simulink model "model_equation"  (R2021a)
settings: Solver=FixedStepAuto  StartTime=0.0  StopTime=10.0  FixedStep=Ts  RelTol=1e-3
undefined symbols (not defined in the file): acc_C, acc_enable, acc_noise_var, B_hs, b_large_bot, b_large_up, b_small_bot, b_small_up, bot_damp_start, C_1, C_2, C_A_in, C_A_out, C_adj_in, C_adj_out, C_B_in, C_B_out, cycle, F_c, F_df, F_sf, flow_C, flow_C_ratio, flow_noise_var, g, gamma, gn, gp, K_hs, k_small_bot, k_small_up, L, LargeDamper_bottom, LargeDamper_upper, M, M_L, p0, p1, p2, p3, p4, P_0, p_A0, p_B0, P_cr, P_s, prox_bot_band, prox_up_band, R, S_0, S_A, S_B, sg_C, sg_enable, sg_noise_var, SmallDamper_bottom, SmallDamper_upper, spool_dynamic, spool_valve_time_delay, T ... (+6)
settings Model: OrderedModelArguments=off  Creator=artof  LastModifiedBy=artof
settings DataIOCC: ExternalInput=[t, u1, u2]  LoadExternalInput=on

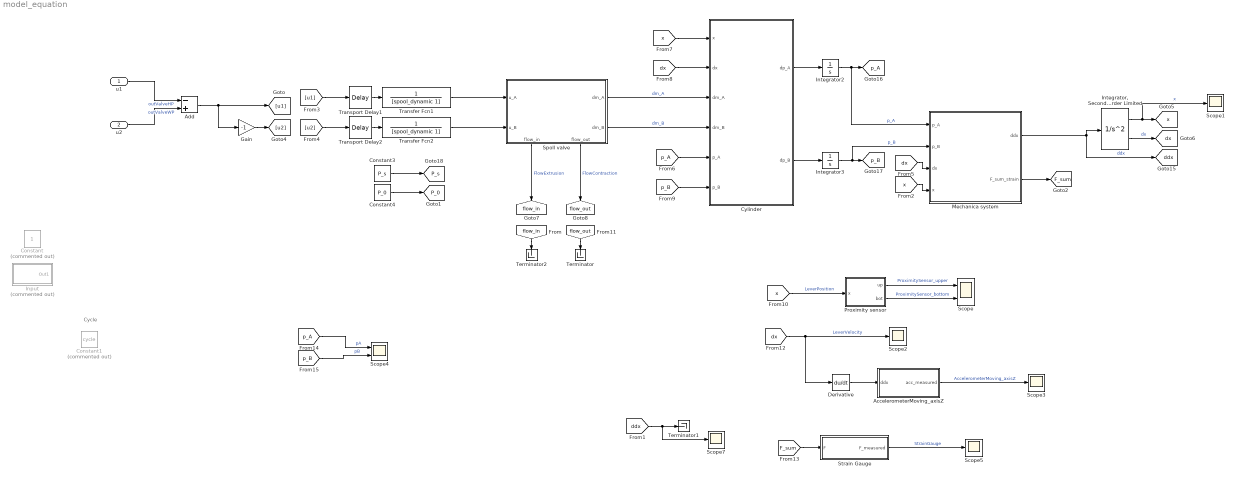
== system model_equation ==
  note: Cycle
  u1 : Inport
  u2 : Inport  Port=2
  AccelerometerMoving_axisZ : MATLAB Function  TreatAsAtomicUnit=on
  Add : Sum  Inputs=-+
  Constant : Constant  Commented=on
  Constant1 : Constant  Commented=on  Value=cycle  VectorParams1D=off  OutDataTypeStr=double
  Constant3 : Constant  Value=P_s
  Constant4 : Constant  Value=P_0
  Cylinder : MATLAB Function  TreatAsAtomicUnit=on
  Derivative : Derivative
  Gain : Gain  Gain=-1
  Input : Subsystem  Commented=on
  "Integrator, Second-Order Limited" : SecondOrderIntegrator  ICX=x0  UpperLimitX=gp  LowerLimitX=gn
  Integrator2 : Integrator  InitialCondition=p_A0
  Integrator3 : Integrator  InitialCondition=p_B0
  Mechanica system : MATLAB Function  TreatAsAtomicUnit=on
  Proximity sensor : MATLAB Function  TreatAsAtomicUnit=on
  Scope : Scope  NumInputPorts=2
  Scope{1..3,5,7} (5 alike) : Scope
  Scope4 : Scope  NumInputPorts=2
  Spoll valve : Subsystem
      settings: PortSchema="{\"entries\":[{\"content\":{\"sides\":[{\"content\":{\"connectorIds\":[\"In1\",\"In2\"]},\"type\":\"ConnectorPlacement.EquallySpacedRectSide\",\"uuid\":\"f49fadee-fa9e-4c00-be17-3013d1757a7f\"},{\"content\":{\"connectorIds\":[\"Out1\",\"Out2\"],\"side\":\"RIGHT\"},\"type\":\"ConnectorPlacement.EquallySpacedRectSide\",\"uuid\":\"640b0073-0df7-45c7-9e72-cb244187d5a1\"},{\"content\":{\"connectorIds\":[],\"side\":\"TOP\"},\"type\":\"ConnectorPlacement.EquallySpacedRectSide\",\"uuid\":\"42e207d6-f026-4ddf-97dc-8c7968fc41f1\"},{\"content\":{\"connectorIds\":[\"Out3\",\"Out4\"],\"side\":\"BOTTOM\"},\"type\":\"ConnectorPlacement.EquallySpacedRectSide\",\"uuid\":\"eeba3cdd-6d70-46a7-a1e2-c2998fe430fd\"}]},\"type\":\"ConnectorPlacement.EquallySpacedConnector\",\"uuid\":\"e8c5a427-dc83-42b8-9540-729b85904a46\"}],\"packageUris\":[\"http://schema.mathworks.com/mf0/Connector/R2020b\"],\"version\":\"1.0\"}"
  Strain Gauge : MATLAB Function  TreatAsAtomicUnit=on
  Terminator : Terminator
  Terminator1 : Terminator
  Terminator2 : Terminator
  Transfer Fcn1 : TransferFcn  Denominator=[spool_dynamic 1]
  Transfer Fcn2 : TransferFcn  Denominator=[spool_dynamic 1]
  Transport Delay1 : TransportDelay  DelayTime=spool_valve_time_delay
  Transport Delay2 : TransportDelay  DelayTime=spool_valve_time_delay
  tag scope: F_sum=global, P_0=global, P_s=global, ddx=global, dx=global, flow_in=global, flow_out=global, p_A=global, p_B=global, x=global
  wires:
  Integrator2/1 -> Mechanica system/1(p_A), [p_A]  "p_A"
  Transport Delay2/1 -> Transfer Fcn2/1
  u1/1 -> Add/1  "outValveHP"
  "Integrator, Second-Order Limited"/1 -> Scope1/1, [x]  "x"
  [x] -> Mechanica system/4(x)
  Proximity sensor/2(bot) -> Scope/2  "ProximitySensor_bottom"
  [flow_out] -> Terminator/1
  Proximity sensor/1(up) -> Scope/1  "ProximitySensor_upper"
  [u2] -> Transport Delay2/1
  Transfer Fcn2/1 -> Spoll valve/2(u_B)
  Spoll valve/1(dm_A) -> Cylinder/3(dm_A)  "dm_A"
  Transfer Fcn1/1 -> Spoll valve/1(u_A)
  [ddx] -> Scope7/1, Terminator1/1
  [p_A] -> Cylinder/5(p_A)
  Spoll valve/4(flow_out) -> [flow_out]  "FlowContraction"
  [F_sum] -> Strain Gauge/1(F)
  Strain Gauge/1(F_measured) -> Scope5/1  "StrainGauge"
  Spoll valve/2(dm_B) -> Cylinder/4(dm_B)  "dm_B"
  [flow_in] -> Terminator2/1
  Mechanica system/1(ddx) -> "Integrator, Second-Order Limited"/1, [ddx]  "ddx"
  Integrator3/1 -> Mechanica system/2(p_B), [p_B]  "p_B"
  Constant3/1 -> [P_s]
  [dx] -> Derivative/1, Scope2/1  "LeverVelocity"
  Transport Delay1/1 -> Transfer Fcn1/1
  Gain/1 -> [u2]
  Constant4/1 -> [P_0]
  Cylinder/1(dp_A) -> Integrator2/1
  Mechanica system/2(F_sum_strain) -> [F_sum]
  [p_B] -> Cylinder/6(p_B)
  Derivative/1 -> AccelerometerMoving_axisZ/1(ddx)
  [dx] -> Mechanica system/3(dx)
  [u1] -> Transport Delay1/1
  AccelerometerMoving_axisZ/1(acc_measured) -> Scope3/1  "AccelerometerMoving_axisZ"
  Cylinder/2(dp_B) -> Integrator3/1
  [dx] -> Cylinder/2(dx)
  [x] -> Cylinder/1(x)
  Spoll valve/3(flow_in) -> [flow_in]  "FlowExtrusion"
  Add/1 -> Gain/1, [u1]
  "Integrator, Second-Order Limited"/2 -> [dx]  "dx"
  [x] -> Proximity sensor/1(x)  "LeverPosition"
  u2/1 -> Add/2  "outValveWP"
  [p_B] -> Scope4/2  "pB"
  [p_A] -> Scope4/1  "pA"

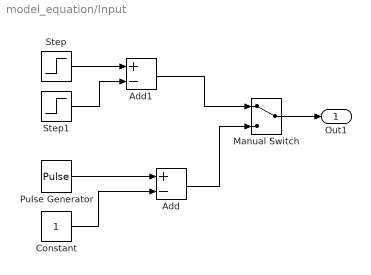
== system model_equation/Input ==
  Add : Sum  Inputs=+-
  Add1 : Sum  Inputs=+-
  Constant : Constant
  Manual Switch : ManualSwitch
  Pulse Generator : DiscretePulseGenerator  PulseType=Time based  Amplitude=2  Period=10  PulseWidth=50
  Step : Step  Before=-1  SampleTime=0
  Step1 : Step  Time=6  After=2  SampleTime=0
  Out1 : Outport
  wires:
  Manual Switch/1 -> Out1/1
  Add/1 -> Manual Switch/2
  Add1/1 -> Manual Switch/1
  Pulse Generator/1 -> Add/1
  Constant/1 -> Add/2
  Step1/1 -> Add1/2
  Step/1 -> Add1/1

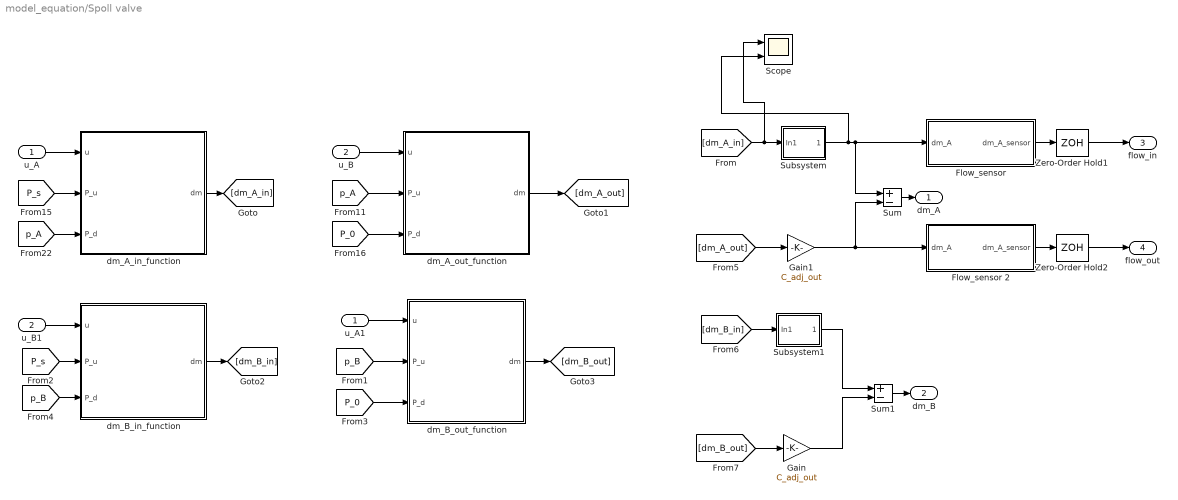
== system model_equation/Spoll valve ==
  u_A : Inport
  u_B : Inport  Port=2
  Flow_sensor : MATLAB Function  TreatAsAtomicUnit=on
  Flow_sensor 2 : MATLAB Function  TreatAsAtomicUnit=on
  Gain : Gain  Gain=C_adj_out
  Gain1 : Gain  Gain=C_adj_out
  Scope : Scope  NumInputPorts=2
  Subsystem : Subsystem
  Subsystem1 : Subsystem
  Sum : Sum  Inputs=+-
  Sum1 : Sum  Inputs=+-
  Zero-Order Hold1 : ZeroOrderHold  SampleTime=Ts
  Zero-Order Hold2 : ZeroOrderHold  SampleTime=Ts
  dm_A_in_function : MATLAB Function  TreatAsAtomicUnit=on
  dm_A_out_function : MATLAB Function  TreatAsAtomicUnit=on
  dm_B_in_function : MATLAB Function  TreatAsAtomicUnit=on
  dm_B_out_function : MATLAB Function  TreatAsAtomicUnit=on
  u_A1 : InportShadow
  u_B1 : InportShadow  Port=2
  dm_A : Outport
  dm_B : Outport  Port=2
  flow_in : Outport  Port=3
  flow_out : Outport  Port=4
  wires:
  [P_s] -> dm_A_in_function/2(P_u)
  [p_A] -> dm_A_in_function/3(P_d)
  dm_A_in_function/1(dm) -> [dm_A_in]
  dm_A_out_function/1(dm) -> [dm_A_out]
  [p_A] -> dm_A_out_function/2(P_u)
  [P_0] -> dm_A_out_function/3(P_d)
  u_A/1 -> dm_A_in_function/1(u)
  u_B/1 -> dm_A_out_function/1(u)
  u_B1/1 -> dm_B_in_function/1(u)
  [P_0] -> dm_B_out_function/3(P_d)
  [p_B] -> dm_B_out_function/2(P_u)
  [p_B] -> dm_B_in_function/3(P_d)
  [P_s] -> dm_B_in_function/2(P_u)
  u_A1/1 -> dm_B_out_function/1(u)
  dm_B_in_function/1(dm) -> [dm_B_in]
  dm_B_out_function/1(dm) -> [dm_B_out]
  [dm_A_in] -> Subsystem/1(In1), Scope/1
  Sum/1 -> dm_A/1
  Sum1/1 -> dm_B/1
  [dm_B_out] -> Gain/1
  [dm_B_in] -> Subsystem1/1(In1)
  Flow_sensor/1(dm_A_sensor) -> Zero-Order Hold1/1
  Flow_sensor 2/1(dm_A_sensor) -> Zero-Order Hold2/1
  [dm_A_out] -> Gain1/1
  Zero-Order Hold1/1 -> flow_in/1
  Zero-Order Hold2/1 -> flow_out/1
  Subsystem1/1(Out1) -> Sum1/1
  Subsystem/1(Out1) -> Scope/2, Sum/1, Flow_sensor/1(dm_A)
  Gain/1 -> Sum1/2
  Gain1/1 -> Flow_sensor 2/1(dm_A), Sum/2

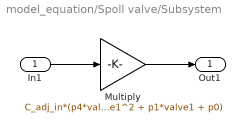
== system model_equation/Spoll valve/Subsystem ==
  In1 : Inport
  Multiply : Gain  Gain=C_adj_in*(p4*valve1^4 + p3*valve1^3+p2*valve1^2 + p1*valve1 + p0)
  Out1 : Outport
  wires:
  In1/1 -> Multiply/1
  Multiply/1 -> Out1/1

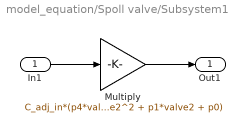
== system model_equation/Spoll valve/Subsystem1 ==
  In1 : Inport
  Multiply : Gain  Gain=C_adj_in*(p4*valve2^4 + p3*valve2^3+p2*valve2^2 + p1*valve2 + p0)
  Out1 : Outport
  wires:
  Multiply/1 -> Out1/1
  In1/1 -> Multiply/1

== matlab function model_equation/Cylinder ==
  data: x input; dp_A output size=1; dx input; dm_A input; dm_B input; p_A input; p_B input; gamma parameter; V_0A parameter; V_0B parameter; S_A parameter; S_B parameter; R parameter; T parameter; dp_B output size=1; L parameter
function [dp_A,dp_B]= fcn(x,dx,dm_A,dm_B,p_A,p_B,gamma,V_0A,V_0B,S_A,S_B,R,T,L)
V_A = V_0A + S_A*x;
dV_A = dx * S_A;

V_B = V_0B + S_B*(L-x);
dV_B = - dx * S_B;

dp_A = dm_A*gamma*R*T/V_A - p_A*gamma*dV_A/V_A;
dp_B = dm_B*gamma*R*T/V_B - p_B*gamma*dV_B/V_B;
end

== matlab function model_equation/Spoll valve/dm_A_in_function ==
  data: u input; dm output; P_u input; P_d input; C_A_in parameter; C_1 parameter; C_2 parameter; P_cr parameter; T parameter; gamma parameter
function dm = fcn(u, P_u, P_d, C_A_in, C_1, C_2, P_cr, T, gamma)
if u > 0    
    P_ratio = P_d/P_u;
    if P_ratio <= P_cr && P_ratio >= 0
        dm = u*C_A_in*C_1*P_u/sqrt(T);
    elseif P_ratio > P_cr && P_ratio <= 1
        dm = u*C_A_in*C_2*P_u/sqrt(T)*P_ratio^(1/gamma)*sqrt(1-P_ratio^((gamma-1)/gamma));
    else
        %dm = -u*C_A_in*C_2*P_d/sqrt(T)*(1/P_ratio)^(1/gamma)*sqrt(1-(1/P_ratio)^((gamma-1)/gamma));
        dm = 0;
    end
else
    dm = 0;
end

== matlab function model_equation/Spoll valve/dm_A_out_function ==
  data: u input; dm output; P_u input; P_d input; C_A_out parameter; C_1 parameter; P_cr parameter; C_2 parameter; T parameter; gamma parameter
function dm = fcn(u, P_u, P_d, C_A_out, C_1, P_cr, C_2, T, gamma)
if u > 0    
    P_ratio = P_d/P_u;
    if P_ratio <= P_cr && P_ratio >= 0
        dm = u*C_A_out*C_1*P_u/sqrt(T);
    elseif P_ratio > P_cr && P_ratio <= 1
        dm = u*C_A_out*C_2*P_u/sqrt(T)*P_ratio^(1/gamma)*sqrt(1-P_ratio^((gamma-1)/gamma));
    else
        %dm = -u*C_A_out*C_2*P_d/sqrt(T)*(1/P_ratio)^(1/gamma)*sqrt(1-(1/P_ratio)^((gamma-1)/gamma));
        dm = 0;
    end
else
    dm = 0;
end

== matlab function model_equation/Spoll valve/dm_B_in_function ==
  data: u input; dm output; P_u input; P_d input; P_cr parameter; C_B_in parameter; C_1 parameter; C_2 parameter; T parameter; gamma parameter
function dm = fcn(u, P_u, P_d, P_cr, C_B_in, C_1, C_2, T, gamma)
if u > 0    
    P_ratio = P_d/P_u;
    if P_ratio <= P_cr && P_ratio >= 0
        dm = u*C_B_in*C_1*P_u/sqrt(T);
    elseif P_ratio > P_cr && P_ratio <= 1
        dm = u*C_B_in*C_2*P_u/sqrt(T)*P_ratio^(1/gamma)*sqrt(1-P_ratio^((gamma-1)/gamma));
    else
        %dm = -u*C_B_in*C_2*P_d/sqrt(T)*(1/P_ratio)^(1/gamma)*sqrt(1-(1/P_ratio)^((gamma-1)/gamma));
        dm = 0;
    end
else
    dm = 0;
end

== matlab function model_equation/Spoll valve/dm_B_out_function ==
  data: u input; dm output; P_u input; P_d input; P_cr parameter; C_B_out parameter; C_1 parameter; C_2 parameter; T parameter; gamma parameter
function dm = fcn(u, P_u, P_d, P_cr, C_B_out, C_1, C_2, T, gamma)
if u > 0    
    P_ratio = P_d/P_u;
    if P_ratio <= P_cr && P_ratio >= 0
        dm = u*C_B_out*C_1*P_u/sqrt(T);
    elseif P_ratio > P_cr && P_ratio <= 1
        dm = u*C_B_out*C_2*P_u/sqrt(T)*P_ratio^(1/gamma)*sqrt(1-P_ratio^((gamma-1)/gamma));
    else
        %dm = -u*C_B_out*C_2*P_d/sqrt(T)*(1/P_ratio)^(1/gamma)*sqrt(1-(1/P_ratio)^((gamma-1)/gamma));
        dm = 0;
    end
else
    dm = 0;
end

== matlab function model_equation/AccelerometerMoving_axisZ ==
  settings: updateMethod=DISCRETE  sampleTime=Ts
  data: ddx input; acc_measured output; acc_noise_var parameter; acc_enable parameter; acc_C parameter
function acc_measured = fcn(ddx, acc_noise_var, acc_enable, acc_C)

ZeroOffset = 2.5; % V
Sensetivity = 333; %mv/g

acc = acc_enable * acc_C * ddx + 1;

U_raw = acc*Sensetivity/1000 + ZeroOffset;
U_raw = U_raw + acc_noise_var*(2*rand()-1);

acc_measured =  acc_enable*((U_raw - ZeroOffset)*1000/Sensetivity);
end

== matlab function model_equation/Proximity sensor ==
  data: x input; up output; bot output; prox_up_band parameter; prox_bot_band parameter
function [up,bot]= fcn(x, prox_up_band, prox_bot_band)
if x >= prox_up_band
    up = 1; bot = 0;
elseif x <= prox_bot_band
    bot = 1; up = 0;
else
    bot = 0;
    up = 0;
end

== matlab function model_equation/Spoll valve/Flow_sensor ==
  settings: updateMethod=DISCRETE
  data: dm_A input; dm_A_sensor output; flow_C parameter; flow_C_ratio parameter; flow_noise_var parameter
function dm_A_sensor = fcn(dm_A, flow_C, flow_C_ratio, flow_noise_var)
dm_A_sensor = flow_C*(flow_C_ratio*dm_A + flow_noise_var*(2*rand()-1));
end

== matlab function model_equation/Spoll valve/Flow_sensor 2 ==
  settings: updateMethod=DISCRETE
  data: dm_A input; dm_A_sensor output; flow_C parameter; flow_C_ratio parameter; flow_noise_var parameter
function dm_A_sensor = fcn(dm_A, flow_C, flow_C_ratio, flow_noise_var)
dm_A_sensor = flow_C*(flow_C_ratio*dm_A + flow_noise_var*(2*rand()-1));

== matlab function model_equation/Strain Gauge ==
  settings: updateMethod=DISCRETE
  data: F input; F_measured output; sg_enable parameter; sg_noise_var parameter; sg_C parameter
function F_measured = fcn(F,sg_enable, sg_noise_var, sg_C)
U = sg_enable*(sg_C*F + sg_noise_var*(2*rand()-1));
F_measured = U*1/sg_C;
end

== matlab function model_equation/Mechanica system ==
  data: p_A input; ddx output; p_B input; dx input; x input; S_A parameter; S_B parameter; M parameter; M_L parameter; P_0 parameter; S_0 parameter; g parameter; up_damp_start parameter; bot_damp_start parameter; b_small_up parameter; k_small_up parameter; b_small_bot parameter; k_small_bot parameter; SmallDamper_bottom parameter; SmallDamper_upper parameter; F_sum_strain output; K_hs parameter; B_hs parameter; gp parameter; gn parameter; b_large_bot parameter; b_large_up parameter; LargeDamper_bottom parameter; LargeDamper_upper parameter; F_sf parameter; F_df parameter; F_c parameter
function [ddx, F_sum_strain] = fcn(p_A,p_B,dx,x,S_A,S_B,M,M_L,P_0,S_0,g, ...
    up_damp_start,bot_damp_start,b_small_up,k_small_up,b_small_bot,k_small_bot,SmallDamper_bottom,SmallDamper_upper, ...
    K_hs,B_hs,gp,gn,b_large_bot, b_large_up, LargeDamper_bottom, LargeDamper_upper, F_sf, F_df, F_c)



% % Hard Stop
if 1
up_force = K_hs*(x-gp) + B_hs*dx*ge(dx,0);
bot_force = K_hs*(x-gn) + B_hs*dx*le(dx,0);
% up_force = K_hs*(x-gp) + B_hs*dx*abs(x-gp);
% bot_force = K_hs*(x-gn) + B_hs*dx*abs(x-gn);

% Dead zone calculating Hard Stop
if x >= gp
    F_hs = up_force;
elseif x > gn
    F_hs = 0;
else
    F_hs = bot_force;
end

else
F_hs = 0;
end
% Pneumatic equation
F_pneum = p_A*S_A - p_B*S_B - P_0*S_0;

% Viscous Force
% beta1 = beta + 0.001;
% F_f = dx*beta1;
% F_f = sign(dx) * (1 * abs(dx) + 1);
if dx == 0
    F_sd = F_sf;
else
    F_sd = 0;
end
F_f = F_df*dx + F_c*sign(dx) + F_sd;



% Dead zone calculating Small Dampers
up_force = k_small_up*(x-up_damp_start) + SmallDamper_upper*b_small_up*dx*ge(dx,0);
bot_force = k_small_bot*(x-bot_damp_start) + SmallDamper_bottom*b_small_bot*dx*le(dx,0);

if x >= up_damp_start
    F_damp_small = up_force;
elseif x > bot_damp_start
    F_damp_small = 0;
else
    F_damp_small = bot_force;
end


% Dead zone calculating Small Dampers
up_force =  LargeDamper_upper*b_large_up*dx*ge(dx,0);
bot_force =  LargeDamper_bottom*b_large_bot*dx*le(dx,0);

if x >= up_damp_start
    F_damp_large = up_force;
elseif x > bot_damp_start
    F_damp_large = 0;
else
    F_damp_large = bot_force;
end

F_damp = F_damp_small + F_damp_large;

% Gravity
F_g = (M + M_L)*g;

F_sum_strain = F_pneum - F_g;
F_sum = (F_pneum - F_f - F_hs - F_g - F_damp);
% Full mechincal equation
ddx = 1/(M+M_L)*F_sum;
end
